simulink library "ecrobot_nxt_lib"  (Simulink 6.4)
undefined symbols (not defined in the file or in its folder): BatteryVoltage, clearNXTSignalObjects, CompassSensorS1, EnterButton, GyroSensorS1, InitAccessorBlock, InitInterfaceBlock, LightSensorS1, RevolutionSensorA, RunButton, ServoMotorA, set_fcncallname, sfunxymap2, SoundSensorS1, SoundWAV, SystemClock, TouchSensorS1, TRACK_MAP, UltrasonicSensorS1
(part 2 of 2)

== system ecrobot_nxt_lib/Sound WAV Write ==
  In1 : Inport
  Data Store Write : DataStoreWrite  DataStoreName=SoundWAV  SampleTime=-1
  wires:
  In1/1 -> Data Store Write/1

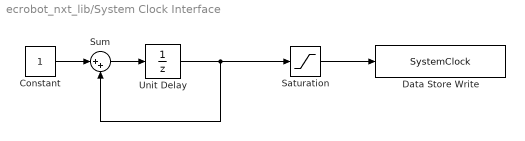
== system ecrobot_nxt_lib/System Clock Interface ==
  Constant : Constant  Value=1  OutDataTypeMode=uint32  OutDataType=sfix(16)  ConRadixGroup=Use specified scaling  OutScaling=2^0  SampleTime=inf  FramePeriod=inf
  Data Store Write : DataStoreWrite  DataStoreName=SystemClock  SampleTime=0.001
  Saturation : Saturate  UpperLimit=SystemClock.Max  LowerLimit=SystemClock.Min  SampleTime=0.001
  Sum : Sum  Inputs=|++  OutDataTypeMode=uint32
  Unit Delay : UnitDelay  SampleTime=0.001
  wires:
  Constant/1 -> Sum/1
  Sum/1 -> Unit Delay/1
  Saturation/1 -> Data Store Write/1
  Unit Delay/1 -> Saturation/1, Sum/2

== system ecrobot_nxt_lib/System Clock Read ==
  Data Store Read : DataStoreRead  DataStoreName=SystemClock  SampleTime=-1
  Out1 : Outport
  wires:
  Data Store Read/1 -> Out1/1  "SystemClock_"

== system ecrobot_nxt_lib/Touch Sensor Interface ==
  In1 : Inport
  Data Store Write : DataStoreWrite  DataStoreName=TouchSensorS1  SampleTime=0.001
  Saturation : Saturate  UpperLimit=TouchSensorS1.Max  LowerLimit=TouchSensorS1.Min  SampleTime=0.001
  wires:
  In1/1 -> Saturation/1
  Saturation/1 -> Data Store Write/1

== system ecrobot_nxt_lib/Touch Sensor Read ==
  Data Store Read : DataStoreRead  DataStoreName=TouchSensorS1  SampleTime=-1
  Out1 : Outport
  wires:
  Data Store Read/1 -> Out1/1  "TouchSensor_S1"

== system ecrobot_nxt_lib/USB Rx Interface ==
  In1 : Inport
  S-Function : S-Function  FunctionName=sfun_usb_rx  Parameters=0.001,0,bd_mode
      mask init:
      | bd_mode = InitDeviceSFunBlock(bdroot);
  Saturation : Saturate  UpperLimit=255  LowerLimit=0
  wires:
  In1/1 -> Saturation/1
  Saturation/1 -> S-Function/1

== system ecrobot_nxt_lib/USB Tx Interface ==
  S-Function : S-Function  FunctionName=sfun_usb_tx  Parameters=0.001,0,bd_mode
      mask init:
      | bd_mode = InitDeviceSFunBlock(bdroot);
  Saturation : Saturate  UpperLimit=255  LowerLimit=0
  Out1 : Outport
  wires:
  S-Function/1 -> Saturation/1
  Saturation/1 -> Out1/1

== system ecrobot_nxt_lib/Ultrasonic Sensor Interface ==
  In1 : Inport
  Data Store Write : DataStoreWrite  DataStoreName=UltrasonicSensorS1  SampleTime=0.001
  Saturation : Saturate  UpperLimit=UltrasonicSensorS1.Max  LowerLimit=UltrasonicSensorS1.Min  SampleTime=0.001
  wires:
  In1/1 -> Saturation/1
  Saturation/1 -> Data Store Write/1

== system ecrobot_nxt_lib/Ultrasonic Sensor Read ==
  Data Store Read : DataStoreRead  DataStoreName=UltrasonicSensorS1  SampleTime=-1
  Out1 : Outport
  wires:
  Data Store Read/1 -> Out1/1  "UltrasonicSensor_S1"

== system ecrobot_nxt_lib/Utilities for simulation ==
  XY Map Graph : Subsystem  LoadFcn=sfunxymap2([],[],[],'LoadBlock')  StartFcn=sfunxymap2([],[],[],'Start')  StopFcn=sfunxymap2([],[],[],'Stop')  TreatAsAtomicUnit=on  SimViewingDevice=on  mask(XYMAP scope.){xmin=0, xmax=200, ymin=0, ymax=200, map=TRACK_MAP}
      mask prompts: xmin "x-min:"; xmax "x-max:"; ymin "y-min:"; ymax "y-max:"; map "track map:"
      mask help: Plots second input (Y) against first input (X) at each time step to create an X-Y plot. Ignores data outside the ranges specified by x-min, x-max, y-min, y-max. bit map file (with '.bmp' extention) image is also plotted in the scope.
      settings: CopyFcn=sfunxymap2([],[],[],'CopyBlock')  DeleteFcn=sfunxymap2([],[],[],'DeleteBlock')  NameChangeFcn=sfunxymap2([],[],[],'NameChange')
      mask Help: This block can be used to explore limit cycles. Look at the m-file sfunxymap.m to see how it works.
      mask Display: plot([.05 .95 .95 .05 .05],[.45 .45 .95 .95 .45], 0.5+cos(0:0.1:2*pi)*0.3,0.7+sin(0:0.1:2*pi)*0.2)

== system ecrobot_nxt_lib/JSP Semaphore/System Outputs ==

== system ecrobot_nxt_lib/JSP Semaphore/System Update ==

== system ecrobot_nxt_lib/OSEK Resource/System Outputs ==

== system ecrobot_nxt_lib/OSEK Resource/System Update ==

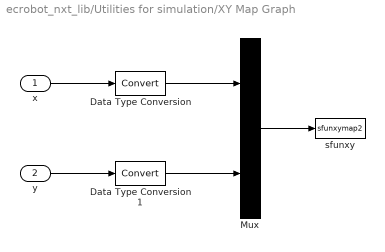
== system ecrobot_nxt_lib/Utilities for simulation/XY Map Graph ==
  x : Inport
  y : Inport  Port=2
  Data Type Conversion : DataTypeConversion  OutDataTypeMode=double
  Data Type Conversion1 : DataTypeConversion  OutDataTypeMode=double
  Mux : Mux  Inputs=2
  sfunxy : S-Function  FunctionName=sfunxymap2  Parameters=[xmin xmax ymin ymax], map
  wires:
  Mux/1 -> sfunxy/1
  x/1 -> Data Type Conversion/1
  y/1 -> Data Type Conversion1/1
  Data Type Conversion/1 -> Mux/1
  Data Type Conversion1/1 -> Mux/2
